simulink model "emldemo_led_switch"  (Simulink 7.6)
settings: Solver=FixedStepDiscrete  StartTime=0.0  StopTime=9  FixedStep=1  RelTol=1e-3
settings Model: Creator=The MathWorks Inc.
settings DebuggingCC: StrictBusMsg=Warning
settings SFSimCC: SimParseCustomCode=off

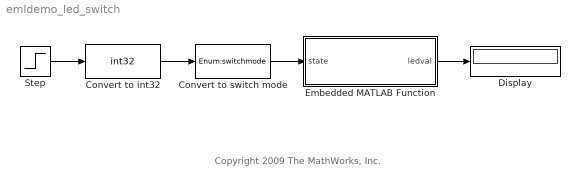
== system emldemo_led_switch ==
  note: Copyright 2009 The MathWorks, Inc.
  Convert to int32 : DataTypeConversion  OutMin=0  OutMax=1  OutDataTypeStr=int32
  Convert to switch mode : DataTypeConversion  OutDataTypeStr=Enum:switchmode  SaturateOnIntegerOverflow=on
  Display : Display
  Embedded MATLAB Function : Stateflow chart  TreatAsAtomicUnit=on
  Step : Step  SampleTime=10
  wires:
  Embedded MATLAB Function/1(ledval) -> Display/1
  Convert to switch mode/1 -> Embedded MATLAB Function/1(state)
  Step/1 -> Convert to int32/1
  Convert to int32/1 -> Convert to switch mode/1

== matlab function Embedded MATLAB Function ==
  data: state input double; ledval output Enum: led
function ledval = checkState(state)
%#eml

if state == switchmode.ON
    ledval = led.GREEN;
else
    ledval = led.RED;
end
